simulink model "DiffBot2014a"  (R2014a)
settings: Solver=ode45  StartTime=0.0  StopTime=5  RelTol=1e-3
values from neighbouring files (symbols this model uses):
  Tstep = 0.01    [RobotControlMain.m]
  x0 = -1    [RobotControlMain.m]
libraries: simulink x1
settings Model: CovHtmlReporting=off  Creator=Gu  LastModifiedBy=duong
settings DataIOCC: SignalLoggingSaveFormat=ModelDataLogs
settings OptimizationCC: ExpressionDepthLimit=2147483647
settings DebuggingCC: UnderspecifiedInitializationDetection=Classic  SolverPrmCheckMsg=none  FcnCallInpInsideContextMsg=EnableAllAsWarning  FrameProcessingCompatibilityMsg=error  StateNameClashWarn=warning
settings SFSimCC: SimParseCustomCode=off
settings GRTTargetCC: CombineOutputUpdateFcns=off  GRTInterface=on

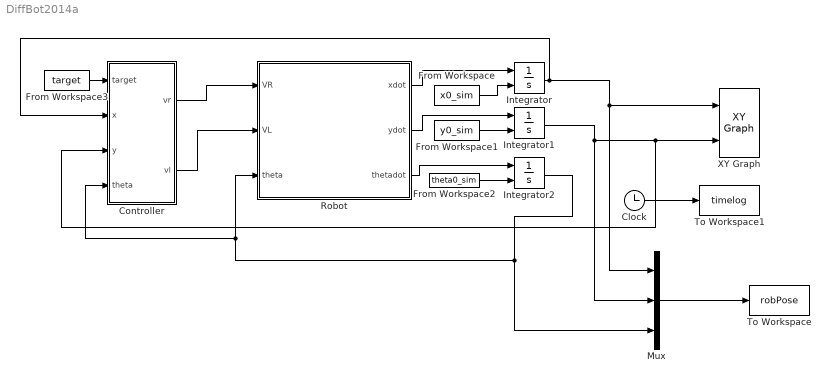
== system DiffBot2014a ==
  Clock : Clock
  Controller : MATLAB Function  TreatAsAtomicUnit=on
      settings: PermitHierarchicalResolution=ParametersOnly
  From Workspace : FromWorkspace  VariableName=x0_sim  OutputAfterFinalValue=Holding final value
  From Workspace1 : FromWorkspace  VariableName=y0_sim  OutputAfterFinalValue=Holding final value
  From Workspace2 : FromWorkspace  VariableName=theta0_sim  OutputAfterFinalValue=Holding final value
  From Workspace3 : FromWorkspace  VariableName=target  OutputAfterFinalValue=Holding final value
  Integrator : Integrator  InitialConditionSource=external  InitialCondition=x0
  Integrator1 : Integrator  InitialConditionSource=external  InitialCondition=2
  Integrator2 : Integrator  InitialConditionSource=external  InitialCondition=pi/4
  Mux : Mux  Inputs=3
  Robot : MATLAB Function  TreatAsAtomicUnit=on
      settings: PermitHierarchicalResolution=ParametersOnly
  To Workspace : ToWorkspace  VariableName=robPose  SampleTime=Tstep
  To Workspace1 : ToWorkspace  VariableName=timelog  SampleTime=-1
      settings: Save2DSignal=2-D array (concatenate along first dimension)
  XY Graph : simulink/Sinks/XY Graph  xmin=-10  xmax=10  ymin=-10  ymax=10  st=-1
  wires:
  Robot/1(xdot) -> Integrator/1
  Robot/2(ydot) -> Integrator1/1
  Robot/3(thetadot) -> Integrator2/1
  Integrator2/1 -> Controller/4(theta), Robot/3(theta), Mux/3
  Integrator/1 -> Controller/2(x), XY Graph/1, Mux/1
  Integrator1/1 -> Controller/3(y), XY Graph/2, Mux/2
  Clock/1 -> To Workspace1/1
  Mux/1 -> To Workspace/1
  From Workspace/1 -> Integrator/2
  From Workspace1/1 -> Integrator1/2
  From Workspace2/1 -> Integrator2/2
  From Workspace3/1 -> Controller/1(target)
  Controller/1(vr) -> Robot/1(VR)
  Controller/2(vl) -> Robot/2(VL)

== matlab function DiffBot2014a/Controller ==
  data: vr output; target input; vl output; x input; y input; theta input
function [vr,vl] = fcn(target,x,y,theta)

% Control parameters
gamma=3;
lamda=6;
h=1;

% Robot parameter: Distance between two wheels
d=0.5;

% Calculate polar variables
rho = sqrt((target(1)-x)^2+(target(2)-y)^2);
phi = atan2(target(2)-y,target(1)-x)-target(3);
alpha = phi+target(3)-theta;

% Calculate control laws
v = gamma*cos(alpha)*rho;
w = lamda*alpha + gamma*cos(alpha)*sin(alpha)/alpha*(alpha+h*phi);

% Calculate Vl and Vr from v and w
vl = (2*v-d*w)/2;
vr = (2*v+d*w)/2;
end

== matlab function DiffBot2014a/Robot ==
  data: VR input; xdot output; VL input; theta input; ydot output; thetadot output
function [xdot, ydot, thetadot] = fcn(VR, VL,theta)

d=0.5; % axial space
xdot=(VR+VL)/2*cos(theta);
ydot=(VR+VL)/2*sin(theta);
thetadot=(VR-VL)/d;
